simulink model "IntegratedMPCcontroller5states"  (R2021a)
settings: Solver=VariableStepAuto  StartTime=0.0  StopTime=30  RelTol=1e-3
libraries: simulink_extras x1
settings Model: Creator=chnwa  LastModifiedBy=chnwa

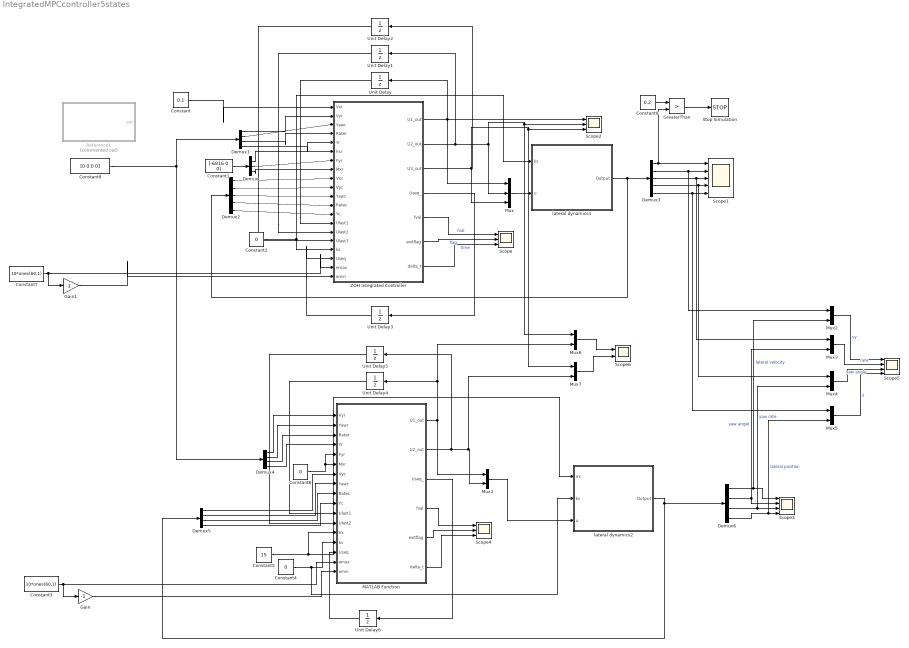
== system IntegratedMPCcontroller5states ==
  Constant : Constant  Value=0.1
  Constant1 : Constant  Value=[-6816 0 0]
  Constant2 : Constant  Value=0
  Constant3 : Constant  Value=10*ones(60,1)
  Constant4 : Constant  Value=0
  Constant5 : Constant  Value=15
  Constant6 : Constant  Value=0
  Constant7 : Constant  Value=10*ones(60,1)
  Constant8 : Constant  Value=[0 0 0 0]
  Constant9 : Constant  Value=0.2
  Demux : Demux  Outputs=3
  Demux{1,4..6} (4 alike) : Demux
  Demux2 : Demux  Outputs=5
  Demux3 : Demux  Outputs=5
  Gain : Gain  Gain=-1
  Gain1 : Gain  Gain=-1
  GreaterThan : RelationalOperator  Operator=>  OutDataTypeStr=boolean  RndMeth=Simplest
  MATLAB Function : MATLAB Function  TreatAsAtomicUnit=on
  Mux : Mux  Inputs=3
  Mux{1..7} (7 alike) : Mux  Inputs=2
  Reference1 : Subsystem  Commented=on  AncestorBlock=Meldas_library/Reference
  Scope : Scope  NumInputPorts=3
  Scope1 : Scope  NumInputPorts=5
  Scope2 : Scope  NumInputPorts=3
  Scope3 : Scope  NumInputPorts=4
  Scope4 : Scope  NumInputPorts=3
  Scope5 : Scope  NumInputPorts=4
  Scope6 : Scope  NumInputPorts=2
  Stop Simulation : Stop
  Unit Delay{,1..2,4..5} (5 alike) : UnitDelay  SampleTime=-1  HasFrameUpgradeWarning=on
  Unit Delay3 : UnitDelay  InitialCondition=[[-6816 0 0];zeros(60,3)]  SampleTime=-1  HasFrameUpgradeWarning=on
  Unit Delay6 : UnitDelay  InitialCondition=zeros(61,2)  SampleTime=-1  HasFrameUpgradeWarning=on
  ZOH Integrated Controller : MATLAB Function  TreatAsAtomicUnit=on
  lateral dynamics1 : Subsystem
  lateral dynamics2 : Subsystem
  wires:
  ZOH Integrated Controller/1(U1_out) -> Mux/1, Unit Delay/1, Scope2/1
  Unit Delay/1 -> ZOH Integrated Controller/14(Ulast1)
  ZOH Integrated Controller/2(U2_out) -> Unit Delay1/1, Mux6/1, Scope2/2, Mux/2
  Unit Delay1/1 -> ZOH Integrated Controller/15(Ulast2)
  ZOH Integrated Controller/3(U3_out) -> Scope2/3, Mux7/1, Mux/3, Unit Delay2/1
  Unit Delay2/1 -> ZOH Integrated Controller/16(Ulast3)
  ZOH Integrated Controller/4(Useq_) -> Unit Delay3/1
  Unit Delay3/1 -> ZOH Integrated Controller/18(Useq)
  Demux1/3 -> ZOH Integrated Controller/4(Rater)
  Demux1/2 -> ZOH Integrated Controller/3(Yawr)
  Demux1/1 -> ZOH Integrated Controller/2(Vyr)
  Demux1/4 -> ZOH Integrated Controller/5(Yr)
  Constant/1 -> ZOH Integrated Controller/1(Vxr)
  Constant1/1 -> Demux/1
  Demux/1 -> ZOH Integrated Controller/6(Fxr)
  Demux/2 -> ZOH Integrated Controller/7(Fyr)
  Demux/3 -> ZOH Integrated Controller/8(Mxr)
  lateral dynamics1/1(Output) -> Demux3/1, Demux2/1
  Demux2/1 -> ZOH Integrated Controller/9(Vxc)
  Demux2/2 -> ZOH Integrated Controller/10(Vyc)
  Demux2/3 -> ZOH Integrated Controller/11(Yawc)
  Demux2/4 -> ZOH Integrated Controller/12(Ratec)
  Demux2/5 -> ZOH Integrated Controller/13(Yc)
  Constant2/1 -> lateral dynamics1/1(ks), ZOH Integrated Controller/17(ks)
  Constant3/1 -> Gain/1, MATLAB Function/16(emax)
  Gain/1 -> MATLAB Function/17(emin)
  Mux/1 -> lateral dynamics1/2(u)
  ZOH Integrated Controller/5(fval) -> Scope/1  "fval"
  ZOH Integrated Controller/6(exitflag) -> Scope/2  "flag"
  ZOH Integrated Controller/7(delta_t) -> Scope/3  "time"
  Demux3/1 -> GreaterThan/2, Scope1/1
  Demux3/2 -> Mux2/1, Scope1/2
  Demux3/3 -> Mux3/1, Scope1/3
  Demux3/4 -> Mux4/1, Scope1/4
  Demux3/5 -> Mux5/1, Scope1/5
  MATLAB Function/6(delta_t) -> Scope4/3
  Demux5/3 -> MATLAB Function/9(Ratec)
  Demux5/1 -> MATLAB Function/7(Vyc)
  Constant6/1 -> MATLAB Function/5(Fyr), MATLAB Function/6(Mxr)
  Demux6/2 -> Mux3/2, Scope3/2  "yaw angel"
  lateral dynamics2/1(Output) -> Demux5/1, Demux6/1
  MATLAB Function/1(U1_out) -> Mux6/2, Unit Delay4/1, Mux1/1
  Unit Delay5/1 -> MATLAB Function/12(Ulast2)
  MATLAB Function/2(U2_out) -> Mux7/2, Mux1/2, Unit Delay5/1
  MATLAB Function/5(exitflag) -> Scope4/2
  Unit Delay6/1 -> MATLAB Function/15(Useq)
  Demux5/2 -> MATLAB Function/8(Yawc)
  Demux5/4 -> MATLAB Function/10(Yc)
  Demux6/1 -> Mux2/2, Scope3/1  "lateral velocity"
  MATLAB Function/4(fval) -> Scope4/1
  Mux1/1 -> lateral dynamics2/3(u)
  Constant8/1 -> Demux1/1, Demux4/1
  Demux4/1 -> MATLAB Function/1(Vyr)
  Constant4/1 -> lateral dynamics2/2(ks), MATLAB Function/14(ks)
  Constant5/1 -> lateral dynamics2/1(Vx), MATLAB Function/13(Vx)
  Demux4/3 -> MATLAB Function/3(Rater)
  MATLAB Function/3(Useq_) -> Unit Delay6/1
  Demux4/2 -> MATLAB Function/2(Yawr)
  Unit Delay4/1 -> MATLAB Function/11(Ulast1)
  Demux6/3 -> Mux4/2, Scope3/3  "yaw rate"
  Demux6/4 -> Mux5/2, Scope3/4  "lateral position"
  Demux4/4 -> MATLAB Function/4(Yr)
  Mux2/1 -> Scope5/1  "vy"
  Mux3/1 -> Scope5/2  "rate"
  Mux4/1 -> Scope5/3  "yaw angle"
  Mux5/1 -> Scope5/4  "y"
  Mux6/1 -> Scope6/1
  Mux7/1 -> Scope6/2
  Constant7/1 -> ZOH Integrated Controller/19(emax), Gain1/1
  Gain1/1 -> ZOH Integrated Controller/20(emin)
  Constant9/1 -> GreaterThan/1
  GreaterThan/1 -> Stop Simulation/1

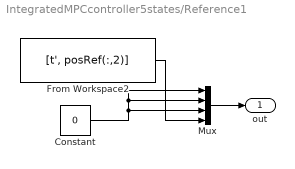
== system IntegratedMPCcontroller5states/Reference1 ==
  Constant : Constant  Value=0
  From Workspace2 : FromWorkspace  VariableName=[t', posRef(:,2)]  SampleTime=0.1
  Mux : Mux
  out : Outport  VectorParamsAs1DForOutWhenUnconnected=off
  wires:
  From Workspace2/1 -> Mux/4
  Constant/1 -> Mux/3, Mux/2, Mux/1
  Mux/1 -> out/1

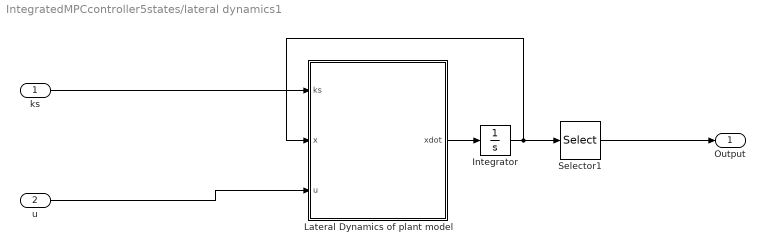
== system IntegratedMPCcontroller5states/lateral dynamics1 ==
  ks : Inport
  u : Inport  Port=2
  Integrator : Integrator  InitialCondition=[15 0 0 0 0]
  Lateral Dynamics of plant model : MATLAB Function  TreatAsAtomicUnit=on
  Selector1 : Selector  InputPortWidth=5  IndexOptions=Index vector (dialog)  Indices=[1 2 3 4 5]  OutputSizes=1
  Output : Outport
  wires:
  u/1 -> Lateral Dynamics of plant model/3(u)
  Lateral Dynamics of plant model/1(xdot) -> Integrator/1
  Integrator/1 -> Selector1/1, Lateral Dynamics of plant model/2(x)
  Selector1/1 -> Output/1
  ks/1 -> Lateral Dynamics of plant model/1(ks)

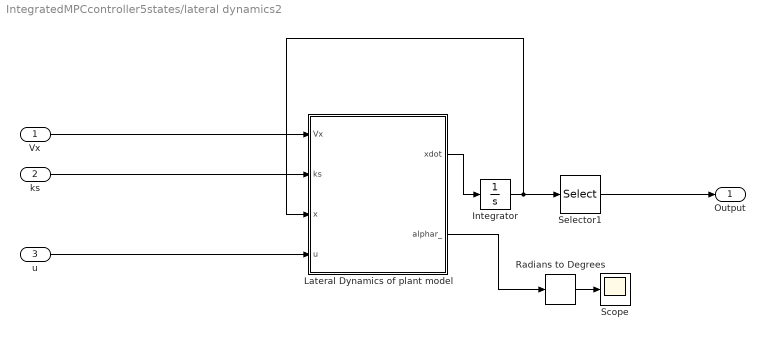
== system IntegratedMPCcontroller5states/lateral dynamics2 ==
  Vx : Inport
  ks : Inport  Port=2
  u : Inport  Port=3
  Integrator : Integrator
  Lateral Dynamics of plant model : MATLAB Function  TreatAsAtomicUnit=on
  Radians to Degrees : simulink_extras/Transformations/Radians to Degrees
  Scope : Scope
  Selector1 : Selector  InputPortWidth=4  IndexOptions=Index vector (dialog)  Indices=[1 2 3 4]  OutputSizes=1
  Output : Outport
  wires:
  u/1 -> Lateral Dynamics of plant model/4(u)
  Lateral Dynamics of plant model/1(xdot) -> Integrator/1
  Integrator/1 -> Selector1/1, Lateral Dynamics of plant model/3(x)
  Selector1/1 -> Output/1
  ks/1 -> Lateral Dynamics of plant model/2(ks)
  Vx/1 -> Lateral Dynamics of plant model/1(Vx)
  Lateral Dynamics of plant model/2(alphar_) -> Radians to Degrees/1
  Radians to Degrees/1 -> Scope/1

== matlab function IntegratedMPCcontroller5states/lateral dynamics2/Lateral Dynamics of plant model ==
  data: Vx input; ks input; x input; u input; xdot output; alphar_ output
function [xdot,alphar_] = fcn(Vx,ks, x, u)

%Plant Model parameters
m = 2272;   %mass
Iz = 4600;  %rotational inertia
lf = 1.11;  % distance from front axle to the mass center
lr = 1.67;  % distance from rear axle to the mass center
C_a = 1.822e5; % rear cornering stifness 

%Enviroment parameters
miu = 0.7; %frction cooeficient 0.7 for dry road and 0.4 for wet
g = 9.81; % gravity

Fz = m*g*lf/(lf+lr); % the load that beared by the rear tire

%calculate alpha
Vy = x(1); %lateral velocity
r = x(2);  %yaw rate
alphar_ = Vy/Vx-lr*r/Vx;   %calculate linearzing point

%tire model
threshold = atan(3*miu*Fz/C_a);
if abs(alphar_)<threshold
    Fyr_ = -C_a*tan(alphar_)+C_a^2/(3*miu*Fz)*abs(tan(alphar_))*tan(alphar_)-C_a^3/(27*miu^2*Fz^2)*tan(alphar_)^3;
    if alphar_>= 0
        Cr_ = -C_a*sec(alphar_)^2+C_a^2/(3*miu*Fz)*(2*sec(alphar_)^2*tan(alphar_))-C_a^3/(27*miu^2*Fz^2)*(3*tan(alphar_)^2*sec(alphar_)^2);
    else
        Cr_ = -C_a*sec(alphar_)^2-C_a^2/(3*miu*Fz)*(2*sec(alphar_)^2*tan(alphar_))-C_a^3/(27*miu^2*Fz^2)*(3*tan(alphar_)^2*sec(alphar_)^2);
    end
else
    Fyr_ = -miu*Fz*sign(alphar_);
    Cr_ = 0;
end

%Continuous-time model
Ac = [Cr_/(m*Vx) -lr*Cr_/(m*Vx)-Vx 0 0;
    -lr*Cr_/(Iz*Vx) lr^2*Cr_/(Iz*Vx) 0 0;
    0 1 0 0;
    1 0 Vx 0];
Bc = [1/m 0;
    lf/Iz 1/Iz;
    0 0;
    0 0];
dcc = [(Fyr_-Cr_*alphar_)/m;
    -lr*(Fyr_-Cr_*alphar_)/Iz;
    -Vx*ks;
    0];

% Cc =eye(4);
% Dc =zeros(4,2);
xdot = Ac*x + Bc*u +dcc;
% y = C*x + D*u;

== matlab function IntegratedMPCcontroller5states/ZOH Integrated Controller ==
  data: Vxr input; Vyr input; U1_out output; Yawr input; Rater input; Yr input; Fxr input; Fyr input; Mxr input; Vxc input; Vyc input; Yawc input; Ratec input; Yc input; Ulast1 input; Ulast2 input; Ulast3 input; ks input; Useq input; U2_out output; U3_out output; Useq_ output; fval output; exitflag output; delta_t output; emax input; emin input
function [U1_out,U2_out,U3_out,Useq_,fval,exitflag,delta_t] = fcn(Vxr,Vyr,Yawr,Rater,Yr, Fxr,Fyr,Mxr,Vxc,Vyc,Yawc,Ratec,Yc,Ulast1,Ulast2,Ulast3,ks,Useq,emax,emin)
%Vyr lateral velocity, Yawr yaw angle, Rater yaw rate, Yr lateral position
%Fyr lateral force in front tyre,Mxr moment generated by longitudinal force
%'r'means reference ||  'c'means current

    tstart=tic;%timing on
    
    if Vxc<0.2
        Vxc=0.2;%make sure many expressions' denominator isn't 0
    end
    lr=1.67;
    threshold=0.1022;
    miu=0.7;
    rmax=9.81*miu/Vxc;
%% Initilization      
    Nx=5;%number of state
    Nu=3;%number of control
    Np=60;%prediction horizon
    Nc=1;%control horizon

    %reference
    r=zeros(Nx,1);%state reference
    r(1)=Vxr;
    r(2)=Vyr;
    r(3)=Yawr;
    r(4)=Rater;
    r(5)=Yr;  
    ur1=Fxr;
    ur2=Fyr;
    ur3=Mxr;%control reference
    
    %states
    x=zeros(Nx,1);%state reference
    x(1)=Vxc;
    x(2)=Vyc;
    x(3)=Yawc;
    x(4)=Ratec;
    x(5)=Yc;   
    
    %control
    u=zeros(Nu,1);%state reference
    u(1)=Ulast1;
    u(2)=Ulast2;
    u(3)=Ulast3;
    
    %get augmented states
    kesi=zeros(Nx+Nu,1);%[X;U]
    kesi(1)=x(1)-r(1);
    kesi(2)=x(2)-r(2);
    kesi(3)=x(3)-r(3);
    kesi(4)=x(4)-r(4);
    kesi(5)=x(5)-r(5);
    kesi(6)=u(1)-ur1;
    kesi(7)=u(2)-ur2;
    kesi(8)=u(3)-ur3;
    
    Ts=0.05;%sample time
    
%% Modellng->Discretization->prediction->quadratic programming
    %Modelling&Linearization&Discretization
    steps=Np+1;
    A = zeros(Nx+Nu,Nx+Nu,steps);
    B = zeros(Nx+Nu,Nu*2,steps);
    Dc = zeros(Nx+Nu,1,steps);
    C=[1 0 0 0 0 0 0 0;0 1 0 0 0 0 0 0;0 0 1 0 0 0 0 0;0 0 0 1 0 0 0 0;0 0 0 0 1 0 0 0];
    
    for ct = 1:steps
        if ct>length(Useq)
            uk = Useq(Np,:);
        else
            uk = Useq(ct,:);
        end
        uk=uk';
        [Ad, Bd, DK, delta_x] = GetDynamics(ks,x,uk,Ts);
        A(:,:,ct)=[Ad,Bd;zeros(Nu,Nx),eye(Nu)];        
        B(:,:,ct)=[Bd zeros(Nx,Nu);eye(Nu) zeros(Nu,Nu)];
        Dc(:,:,ct)=[DK;zeros(Nu,1)];
        x=x+delta_x;    
    end
    %construct important matrix
    %Y=PHI*kesi+THETA*delta_U+OMEGA*D
    coder.varsize('PHI',[Np*Nx,Nx+Nu]);
    coder.varsize('THETA',[Np*Nx,2*Nu]);
    coder.varsize('D',[Np*(Nx+Nu),1]);
    coder.varsize('DD',[Np*Nx,1]);
    PHI=[];
    THETA=zeros(Np*Nx,2*Nu);
    D=[];
    DD=[];
    product=eye(Nx+Nu);
    for j=1:Np
        product=A(:,:,j)*product;
        PHI=[PHI;C*product];
        D=[D;Dc(:,:,j)];
    end
    for k=1:Nc
        product1=eye(Nx+Nu);
        for j=k:Np
            THETA(Nx*(j-1)+1:Nx*j,1:6)=C*product1*B(:,:,Nc);
            product1=A(:,:,j+1)*product1;
        end
    end
    coder.varsize('OMEGA',[Nx*Np,(Nx+Nu)*Np]);
    OMEGA=zeros(Nx*Np,(Nx+Nu)*Np);
    for i=1:Np
        product2=A(:,:,i+1);
        for j=i:Np-1
            if i==j
                OMEGA(Nx*(i-1)+1:Nx*i,(Nx+Nu)*(i-1)+1:(Nx+Nu)*i)=C*eye(Nx+Nu);
            end
            OMEGA(Nx*j+1:Nx*j+Nx,(Nx+Nu)*j+1:(Nx+Nu)*j+(Nx+Nu))=C*product2;
            product2=A(:,:,j+2)*product2;
        end
    end
    DD=OMEGA*D;        
    Sigma=repmat([1 0 0 1 0 0;0 1 0 0 1 0;0 0 1 0 0 1],Np,1);
    Sigma(1:Nu,1:2*Nu)=[1 0 0 0 0 0;0 1 0 0 0 0;0 0 1 0 0 0];
    UT=kron(ones(Np,1),[u(1);u(2);u(3)]);
    error=PHI*kesi;
    Q=kron(eye(Np,Np),diag([4 0 0 100 4]));    
    R=kron(eye(Np,Np),diag([4e-5 0 4e-5]));    
    P=kron(eye(2),diag([0 3e-5 8e-5]));
    rou1=3e3;    
    rou2=5e4;
    H=2*[THETA'*Q*THETA+Sigma'*R*Sigma+P zeros(2*Nu,2);zeros(1,2*Nu) rou1 0;zeros(1,2*Nu) 0 rou2];%是否要乘2？要
    f=[2*(error'*Q*THETA+(OMEGA*D)'*Q*THETA+UT'*R*Sigma),0,0];%是否要转置？好像无所谓
   %% constraints
    %inequation
    A_I=[1 0 0 0 0 0;0 1 0 0 0 0;0 0 1 0 0 0;1 0 0 1 0 0;0 1 0 0 1 0;0 0 1 0 0 1]; 
    Ut=kron(ones(2,1),[Ulast1;Ulast2;Ulast3]);%control in last control step
    umin=[-6816; -1e4; -1e3];
    umax=[6816; 1e4; 1e3];
    Umin=kron(ones(2,1),umin);
    Umax=kron(ones(2,1),umax);
    coder.varsize('A_cons',[Np*6+12,2*Nu+2]);
    coder.varsize('b_cons',[Np*6+12,1]);
    A_cons=[A_I zeros(2*Nu,2);-A_I zeros(2*Nu,2)];
    b_cons=[Umax-Ut;-Umin+Ut];
    %add handling envelop constriants & environment envolop
    gamas=[0 1 -lr 0 0;0 -1 lr 0 0;0 0 1 0 0;0 0 -1 0 0];
    gamae=[0 0 0 0 1;0 0 0 0 -1];
    Gs=[Vxc*threshold;Vxc*threshold;rmax;rmax];
    for i=1:Np
        A_cons=[A_cons;[gamas*THETA(Nx*(i-1)+1:Nx*i,:) -ones(4,1) zeros(4,1)];[gamae*THETA(Nx*(i-1)+1:Nx*i,:) zeros(2,1) -ones(2,1)]];
        b_cons=[b_cons;[Gs-gamas*(PHI(Nx*(i-1)+1:Nx*i,:)*kesi-DD(Nx*(i-1)+1:Nx*i,:))];[emax(i);-emin(i)]-gamae*(PHI(Nx*(i-1)+1:Nx*i,:)*kesi-DD(Nx*(i-1)+1:Nx*i,:))];
    end
    
    %upper and lower boundary
    delta_umin=[-1e4; -1e4; -1e3];
    delta_umax=[1e4; 1e4; 1e3];
    M1=10; %related to slack variable
    M2=10; %related to slack variable
    delta_Umin=kron(ones(2,1),delta_umin);
    delta_Umax=kron(ones(2,1),delta_umax);
    lb=[delta_Umin;0;0];
    ub=[delta_Umax;M1;M2];  
   %% solve quadratic programming
    opts = optimoptions('quadprog','Algorithm','active-set');
    x_start=zeros(Nu*2+2,1);%+2 corresponds to slack variables
    [X,fval,exitflag]=quadprog(H,f',A_cons,b_cons,[],[],lb,ub,x_start,opts);
    
   %% calculate control signal
    U1=kesi(6)+X(1);%The output error at the previous time plus the optimization result to get the error at this time
    U2=kesi(7)+X(2);%The output error at the previous time plus the optimization result to get the error at this time
    U3=kesi(8)+X(3);
    U1_out=U1+ur1;%Error plus reference value to get final output value    
    U2_out=U2+ur2;
    U3_out=U3+ur3;
    Useq_=[U1_out U2_out U3_out; repmat([U1_out+X(4) U2_out+X(5) U3_out+X(6)],Np,1)];
    delta_t=toc(tstart);%timing off
end

function [A, B, DK, delta_x] = GetDynamics(ks,x,u,Ts)

%Plant Model parameters
m = 2272;   %mass
Iz = 4600;  %rotational inertia
lf = 1.11;  % distance from front axle to the mass center
lr = 1.67;  % distance from rear axle to the mass center
C_a = 1.822e5; % rear cornering stiffness 

%Enviroment parameters
miu = 0.7; %frction cooeficient 0.7 for dry road and 0.4 for wet
g = 9.81; % gravity

Fz = m*g*lf/(lf+lr); % the load that beared by the rear tire

%calculate alpha
Vx = x(1); %longitudinal velocity
Vy = x(2); %lateral velocity
r = x(3);  %yaw rate
alphar_ = Vy/Vx-lr*r/Vx;   %calculate linearzing point

%tire model
threshold = atan(3*miu*Fz/C_a);     % threshold for the tire linear region
if abs(alphar_)<threshold
    %the rear lateral force value (f(x0)) at the linearzing point
    Fyr_ = -C_a*tan(alphar_)+C_a^2/(3*miu*Fz)*abs(tan(alphar_))*tan(alphar_)-C_a^3/(27*miu^2*Fz^2)*tan(alphar_)^3;
    
    %the slope of linearized model (f‘(x0))
    if alphar_>= 0
        Cr_ = -C_a*sec(alphar_)^2+C_a^2/(3*miu*Fz)*(2*sec(alphar_)^2*tan(alphar_))-C_a^3/(27*miu^2*Fz^2)*(3*tan(alphar_)^2*sec(alphar_)^2);
    else
        Cr_ = -C_a*sec(alphar_)^2-C_a^2/(3*miu*Fz)*(2*sec(alphar_)^2*tan(alphar_))-C_a^3/(27*miu^2*Fz^2)*(3*tan(alphar_)^2*sec(alphar_)^2);
    end
else
    
    %the saturation region of tire model
    Fyr_ = -miu*Fz*sign(alphar_);
    Cr_ = 0;
end

%Continuous-time model
Ac = [0 r Vy 0 0;
    -r+(Cr_*(lr*r-Vy)/(m*Vx^2)) Cr_/(m*Vx) -lr*Cr_/(m*Vx)-Vx 0 0;
    lr*Cr_*(Vy-lr*r)/(Iz*Vx^2) -lr*Cr_/(Iz*Vx) lr^2*Cr_/(Iz*Vx) 0 0;
    -ks 0 1 0 0;
    0 1 0 Vx 0];
Bc = [1/m 0 0;
    0 1/m 0;
    0 lf/Iz 1/Iz;
    0 0 0;
    0 0 0];
dcc = [0;
    (Fyr_-Cr_*alphar_)/m;
    -lr*(Fyr_-Cr_*alphar_)/Iz;
    -Vx*ks;
    0];
% dcc = dcc-Ac(1:5,1)*Vx;%adjust the Vx's linearization point
G=[Ac Bc dcc;zeros(4,9)];
M=expm(G*Ts);
A=M(1:5,1:5);
B=M(1:5,6:8);
DK=M(1:5,9);
delta_x=A*x+B*u+DK-x;
end

== matlab function IntegratedMPCcontroller5states/MATLAB Function ==
  data: Vyr input; U1_out output; Yawr input; Rater input; Yr input; Fyr input; Mxr input; Vyc input; Yawc input; Ratec input; Yc input; Ulast1 input; Ulast2 input; Vx input; ks input; Useq input; U2_out output; Useq_ output; fval output; exitflag output; delta_t output; emax input; emin input
function [U1_out,U2_out,Useq_,fval,exitflag,delta_t] = fcn(Vyr,Yawr,Rater,Yr, Fyr,Mxr,Vyc,Yawc,Ratec,Yc,Ulast1,Ulast2,Vx,ks,Useq,emax,emin)
%Vyr lateral velocity, Yawr yaw angle, Rater yaw rate, Yr lateral position
%Fyr lateral force in front tyre,Mxr moment generated by longitudinal force
%'r'means reference ||  'c'means current
    if Vx<0.1
        Vx=0.001;%make sure many expressions' denominator isn't 0
    end
    lr=1.67;
    threshold=0.1022;
    miu=0.7;
    rmax=9.81*miu/Vx;
%% Initilization    
    tstart=tic;%timing on
    
    Nx=4;%number of state
    Nu=2;%number of control
    Np=60;%prediction horizon
    Nc=1;%control horizon

    %reference
    r=zeros(Nx,1);%state reference
    r(1)=Vyr;
    r(2)=Yawr;
    r(3)=Rater;
    r(4)=Yr;    
    ur1=Fyr;
    ur2=Mxr;%control reference
    
    %states
    x=zeros(Nx,1);%state reference
    x(1)=Vyc;
    x(2)=Yawc;
    x(3)=Ratec;
    x(4)=Yc;   
    
    %control
    u=zeros(Nu,1);%state reference
    u(1)=Ulast1;
    u(2)=Ulast2;
    
    %get augmented states
    kesi=zeros(Nx+Nu,1);%[X;U]
    kesi(1)=x(1)-r(1);
    kesi(2)=x(2)-r(2);
    kesi(3)=x(3)-r(3);
    kesi(4)=x(4)-r(4);
    kesi(5)=u(1)-ur1;
    kesi(6)=u(2)-ur2;
    
    Ts=0.05;%sample time
    
%% Modellng->Discretization->prediction->quadratic programming
    %Modelling&Linearization&Discretization
    steps=Np+1;
    A = zeros(Nx+Nu,Nx+Nu,steps);
    B = zeros(Nx+Nu,Nu*2,steps);
    Dc = zeros(Nx+Nu,1,steps);
    C=[1 0 0 0 0 0;0 1 0 0 0 0;0 0 1 0 0 0;0 0 0 1 0 0];
    
    for ct = 1:steps
        if ct>length(Useq)
            uk = Useq(Np,:);
        else
            uk = Useq(ct,:);
        end
        uk=uk';
        [Ad, Bd, DK, delta_x] = GetDynamics(Vx,ks,x,uk,Ts);
        A(:,:,ct)=[Ad,Bd;zeros(Nu,Nx),eye(Nu)];        
        B(:,:,ct)=[Bd zeros(4,2);eye(Nu) zeros(2,2)];
        Dc(:,:,ct)=[DK;0;0];
        x=x+delta_x;    
    end
    %construct important matrix
    %Y=PHI*kesi+THETA*delta_U+OMEGA*D
    coder.varsize('PHI',[Np*Nx,Nx+Nu]);
    coder.varsize('THETA',[Np*Nx,2*Nu]);
    coder.varsize('D',[Np*(Nx+Nu),1]);
    coder.varsize('DD',[Np*Nx,1]);
    PHI=[];
    THETA=zeros(Np*Nx,2*Nu);
    D=[];
    DD=[];
    product=eye(6);
    for j=1:Np
        product=A(:,:,j)*product;
        PHI=[PHI;C*product];
        D=[D;Dc(:,:,j)];
    end
    for k=1:Nc
        product1=eye(6);
        for j=k:Np
            THETA(4*j-3:4*j,4*k-3:4*k)=C*product1*B(:,:,Nc);
            product1=A(:,:,j+1)*product1;
        end
    end
    coder.varsize('OMEGA',[Nx*Np,(Nx+Nu)*Np]);
    OMEGA=zeros(Nx*Np,(Nx+Nu)*Np);
    for i=1:Np
        product2=A(:,:,i+1);
        for j=i:Np-1
            if i==j
                OMEGA(4*i-3:4*i,6*i-5:6*i)=C*eye(6);
            end
            OMEGA(4*j+1:4*j+4,6*j+1:6*j+6)=C*product2;
            product2=A(:,:,j+2)*product2;
        end
    end
    DD=OMEGA*D;        
    Sigma=repmat([1 0 1 0;0 1 0 1],Np,1);
    Sigma(1:2,1:4)=[1 0 0 0;0 1 0 0];
    UT=kron(ones(Np,1),[u(1);u(2)]);
    error=PHI*kesi;
    Q=kron(eye(Np,Np),diag([0 0 100 4]));    
    R=kron(eye(Np,Np),diag([0 4e-5]));    
    P=diag([3e-5 8e-5 3e-5 8e-5]);
    rou1=3e3;    
    rou2=5e4;
    H=2*[THETA'*Q*THETA+Sigma'*R*Sigma+P zeros(4,2);zeros(1,4) rou1 0;zeros(1,4) 0 rou2];%是否要乘2？要
    f=[2*(error'*Q*THETA+(OMEGA*D)'*Q*THETA+UT'*R*Sigma),0,0];%是否要转置？好像无所谓
   %% constraints
    %inequation
    A_I=[1 0 0 0;0 1 0 0;1 0 1 0;0 1 0 1]; 
    Ut=kron(ones(2,1),[Ulast1;Ulast2]);%control in last control step
    umin=[-1e4; -1e3];
    umax=[1e4; 1e3];
    Umin=kron(ones(2,1),umin);
    Umax=kron(ones(2,1),umax);
    coder.varsize('A_cons',[Np*6+8,6]);
    coder.varsize('b_cons',[Np*6+8,1]);
    A_cons=[A_I zeros(4,2);-A_I zeros(4,2)];
    b_cons=[Umax-Ut;-Umin+Ut];
    %add handling envelop constriants & environment envolop
    gamas=[1 -lr 0 0;-1 lr 0 0;0 1 0 0;0 -1 0 0];
    gamae=[0 0 0 1;0 0 0 -1];
    Gs=[Vx*threshold;Vx*threshold;rmax;rmax];
    for i=1:Np
        A_cons=[A_cons;[gamas*THETA(4*i-3:4*i,:) -ones(4,1) zeros(4,1)];[gamae*THETA(4*i-3:4*i,:) zeros(2,1) -ones(2,1)]];
        b_cons=[b_cons;[Gs-gamas*(PHI(4*i-3:4*i,:)*kesi-DD(4*i-3:4*i,:))];[emax(i);-emin(i)]-gamae*(PHI(4*i-3:4*i,:)*kesi-DD(4*i-3:4*i,:))];
    end
    
    %upper and lower boundary
    delta_umin=[-1e4;-1e3];
    delta_umax=[1e4;1e3];
    M1=10; %related to slack variable
    M2=10; %related to slack variable
    delta_Umin=kron(ones(2,1),delta_umin);
    delta_Umax=kron(ones(2,1),delta_umax);
    lb=[delta_Umin;0;0];
    ub=[delta_Umax;M1;M2];  
   %% solve quadratic programming
    opts = optimoptions('quadprog','Algorithm','active-set');
    x_start=zeros(Nu*2+2,1);%+2 corresponds to slack variables
    [X,fval,exitflag]=quadprog(H,f',A_cons,b_cons,[],[],lb,ub,x_start,opts);
    
   %% calculate control signal
    U1=kesi(5)+X(1);%The output error at the previous time plus the optimization result to get the error at this time
    U2=kesi(6)+X(2);%The output error at the previous time plus the optimization result to get the error at this time
    U1_out=U1+ur1;%Error plus reference value to get final output value    
    U2_out=U2+ur2;
    Useq_=[U1_out U2_out; repmat([U1_out+X(3) U2_out+X(4)],Np,1)];
    delta_t=toc(tstart);%timing off
end

function [A, B, DK, delta_x] = GetDynamics(Vx,ks,x,u,Ts)

%Plant Model parameters
m = 2272;   %mass
Iz = 4600;  %rotational inertia
lf = 1.11;  % distance from front axle to the mass center
lr = 1.67;  % distance from rear axle to the mass center
C_a = 1.822e5; % rear cornering stiffness 

%Enviroment parameters
miu = 0.7; %frction cooeficient 0.7 for dry road and 0.4 for wet
g = 9.81; % gravity

Fz = m*g*lf/(lf+lr); % the load that beared by the rear tire

%calculate alpha
Vy = x(1); %lateral velocity
r = x(2);  %yaw rate
alphar_ = Vy/Vx-lr*r/Vx;   %calculate linearzing point

%tire model
threshold = atan(3*miu*Fz/C_a);     % threshold for the tire linear region
if abs(alphar_)<threshold
    %the rear lateral force value (f(x0)) at the linearzing point
    Fyr_ = -C_a*tan(alphar_)+C_a^2/(3*miu*Fz)*abs(tan(alphar_))*tan(alphar_)-C_a^3/(27*miu^2*Fz^2)*tan(alphar_)^3;
    
    %the slope of linearized model (f‘(x0))
    if alphar_>= 0
        Cr_ = -C_a*sec(alphar_)^2+C_a^2/(3*miu*Fz)*(2*sec(alphar_)^2*tan(alphar_))-C_a^3/(27*miu^2*Fz^2)*(3*tan(alphar_)^2*sec(alphar_)^2);
    else
        Cr_ = -C_a*sec(alphar_)^2-C_a^2/(3*miu*Fz)*(2*sec(alphar_)^2*tan(alphar_))-C_a^3/(27*miu^2*Fz^2)*(3*tan(alphar_)^2*sec(alphar_)^2);
    end
else
    
    %the saturation region of tire model
    Fyr_ = -miu*Fz*sign(alphar_);
    Cr_ = 0;
end

%Continuous-time model
Ac = [Cr_/(m*Vx) -lr*Cr_/(m*Vx)-Vx 0 0;
    -lr*Cr_/(Iz*Vx) lr^2*Cr_/(Iz*Vx) 0 0;
    0 1 0 0;
    1 0 Vx 0];
Bc = [1/m 0;
    lf/Iz 1/Iz;
    0 0;
    0 0];
dcc = [(Fyr_-Cr_*alphar_)/m;
    -lr*(Fyr_-Cr_*alphar_)/Iz;
    -Vx*ks;
    0];

G=[Ac Bc dcc;zeros(3,7)];
M=expm(G*Ts);
A=M(1:4,1:4);
B=M(1:4,5:6);
DK=M(1:4,7);
delta_x=A*x+B*u+DK-x;
end

== matlab function IntegratedMPCcontroller5states/lateral dynamics1/Lateral Dynamics of plant model ==
  data: ks input; x input; u input; xdot output
function xdot = fcn(ks, x, u)

%Plant Model parameters
m = 2272;   %mass
Iz = 4600;  %rotational inertia
lf = 1.11;  % distance from front axle to the mass center
lr = 1.67;  % distance from rear axle to the mass center
C_a = 1.822e5; % rear cornering stifness 

%Enviroment parameters
miu = 0.7; %frction cooeficient 0.7 for dry road and 0.4 for wet
g = 9.81; % gravity

Fz = m*g*lf/(lf+lr); % the load that beared by the rear tire

%calculate alpha
Vx=x(1);
Vy = x(2); %lateral velocity
r = x(3);  %yaw rate
alphar_ = Vy/Vx-lr*r/Vx;   %calculate linearzing point

%tire model
threshold = atan(3*miu*Fz/C_a);
if abs(alphar_)<threshold
    Fyr_ = -C_a*tan(alphar_)+C_a^2/(3*miu*Fz)*abs(tan(alphar_))*tan(alphar_)-C_a^3/(27*miu^2*Fz^2)*tan(alphar_)^3;
    if alphar_>= 0
        Cr_ = -C_a*sec(alphar_)^2+C_a^2/(3*miu*Fz)*(2*sec(alphar_)^2*tan(alphar_))-C_a^3/(27*miu^2*Fz^2)*(3*tan(alphar_)^2*sec(alphar_)^2);
    else
        Cr_ = -C_a*sec(alphar_)^2-C_a^2/(3*miu*Fz)*(2*sec(alphar_)^2*tan(alphar_))-C_a^3/(27*miu^2*Fz^2)*(3*tan(alphar_)^2*sec(alphar_)^2);
    end
else
    Fyr_ = -miu*Fz*sign(alphar_);
    Cr_ = 0;
end

%Continuous-time model
Ac = [0 r Vy 0 0;
    -r+(Cr_*(lr*r-Vy)/(m*Vx^2)) Cr_/(m*Vx) -lr*Cr_/(m*Vx)-Vx 0 0;
    lr*Cr_*(Vy-lr*r)/(Iz*Vx^2) -lr*Cr_/(Iz*Vx) lr^2*Cr_/(Iz*Vx) 0 0;
    -ks 0 1 0 0;
    0 1 0 Vx 0];
Bc = [1/m 0 0;
    0 1/m 0;
    0 lf/Iz 1/Iz;
    0 0 0;
    0 0 0];
dcc = [0;
    (Fyr_-Cr_*alphar_)/m;
    -lr*(Fyr_-Cr_*alphar_)/Iz;
    -Vx*ks;
    0];

% Cc =eye(4);
% Dc =zeros(4,2);
xdot = Ac*x + Bc*u +dcc;
% y = C*x + D*u;
